simulink model "simple_gain"  (R2021a)
settings: Solver=VariableStepAuto  StartTime=0.0  StopTime=10.0  RelTol=1e-3
settings Model: Creator=Davie  LastModifiedBy=Davie

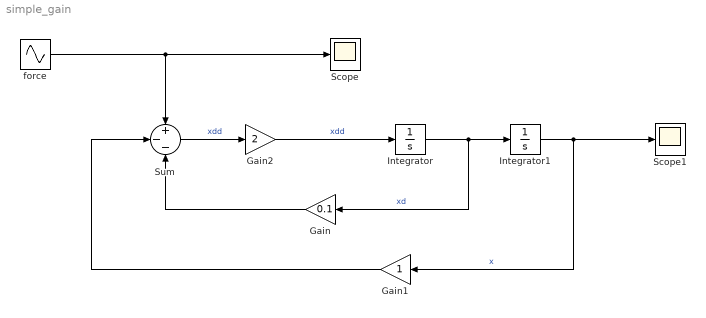
== system simple_gain ==
  Gain : Gain  Gain=0.1
  Gain1 : Gain
  Gain2 : Gain  Gain=2
  Integrator : Integrator
  Integrator1 : Integrator
  Scope : Scope
  Scope1 : Scope
  Sum : Sum  Inputs=+--
  force : Sin  Amplitude=3  SampleTime=0
  wires:
  force/1 -> Sum/1, Scope/1
  Integrator/1 -> Gain/1, Integrator1/1  "xd"
  Sum/1 -> Gain2/1  "xdd"
  Integrator1/1 -> Scope1/1, Gain1/1  "x"
  Gain/1 -> Sum/3
  Gain1/1 -> Sum/2
  Gain2/1 -> Integrator/1  "xdd"
